simulink model "evaluateDis2009b"  (Simulink 7.4)
settings: Solver=ode45  SolverMode=SingleTasking  StartTime=0.0  StopTime=0.4  RelTol=1e-3
values from neighbouring files (symbols this model uses):
  plant = tf(1,[0.01 1])    [transferfunDisObserver_sim.m]
settings Model: Creator=Yu  LastModifiedBy=Yu  CovMetricSettings=dwe  CovHtmlReporting=off  covSaveCumulativeToWorkspaceVar=off  CovSaveSingleToWorkspaceVar=off  CovExternalEMLEnable=on
settings DataIOCC: LimitDataPoints=off  SaveFormat=StructureWithTime
settings OptimizationCC: ExpressionDepthLimit=128
settings DebuggingCC: UnderspecifiedInitializationDetection=Simplified  MergeDetectMultiDrivingBlocksExec=error  SolverPrmCheckMsg=none  FcnCallInpInsideContextMsg=Enable All  StateNameClashWarn=none  StrictBusMsg=ErrorLevel1
settings HardwareCC: ProdIntDivRoundTo=Zero  ProdEndianess=LittleEndian  ProdHWDeviceType=Specified
settings CodeAppCC: CustomSymbolStrType=$N$R$M_T
settings GRTTargetCC: TargetFunctionLibrary=C99 (ISO)  GeneratePreprocessorConditionals=Use local settings

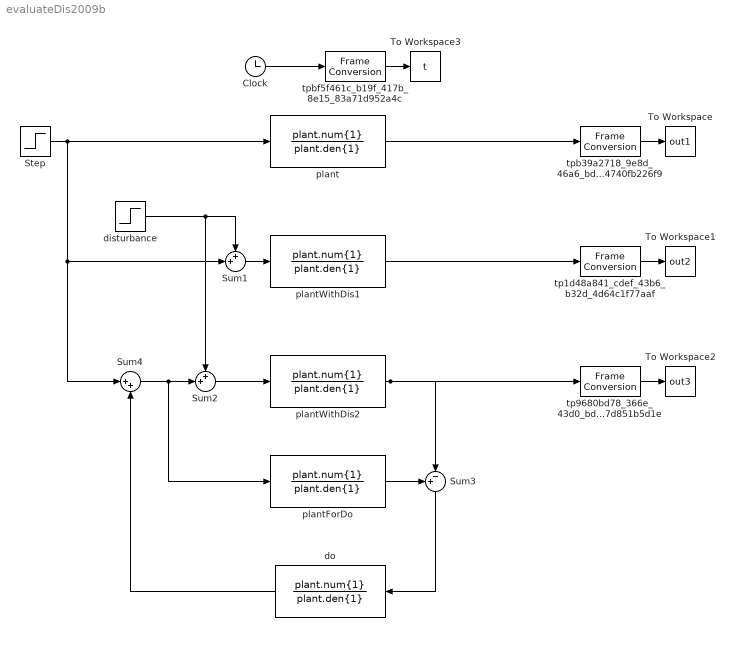
== system evaluateDis2009b ==
  Clock : Clock
  Step : Step  Time=0.01  SampleTime=0
  Sum1 : Sum  Inputs=++|
  Sum2 : Sum  Inputs=++|
  Sum3 : Sum  Inputs=+-|
  Sum4 : Sum  Inputs=|++
  To Workspace : ToWorkspace  VariableName=out1  SampleTime=-1
  To Workspace1 : ToWorkspace  VariableName=out2  SampleTime=-1
  To Workspace2 : ToWorkspace  VariableName=out3  SampleTime=-1
  To Workspace3 : ToWorkspace  VariableName=t  SampleTime=-1
  disturbance : Step  Time=0.2  After=0.3  SampleTime=0
  do : TransferFcn  Numerator=plant.num{1}  Denominator=plant.den{1}
  plant : TransferFcn  Numerator=plant.num{1}  Denominator=plant.den{1}
  plantForDo : TransferFcn  Numerator=plant.num{1}  Denominator=plant.den{1}
  plantWithDis1 : TransferFcn  Numerator=plant.num{1}  Denominator=plant.den{1}
  plantWithDis2 : TransferFcn  Numerator=plant.num{1}  Denominator=plant.den{1}
  tp1d48a841_cdef_43b6_b32d_4d64c1f77aaf : FrameConversion  InheritSamplingMode=off  OutFrame=Sample-based
  tp9680bd78_366e_43d0_bd56_b27d851b5d1e : FrameConversion  InheritSamplingMode=off  OutFrame=Sample-based
  tpb39a2718_9e8d_46a6_bd99_f4740fb226f9 : FrameConversion  InheritSamplingMode=off  OutFrame=Sample-based
  tpbf5f461c_b19f_417b_8e15_83a71d952a4c : FrameConversion  InheritSamplingMode=off  OutFrame=Sample-based
  wires:
  Step/1 -> plant/1, Sum4/1, Sum1/2
  Sum1/1 -> plantWithDis1/1
  Sum2/1 -> plantWithDis2/1
  disturbance/1 -> Sum2/1, Sum1/1
  plantForDo/1 -> Sum3/1
  plantWithDis2/1 -> Sum3/2, tp9680bd78_366e_43d0_bd56_b27d851b5d1e/1
  Sum3/1 -> do/1
  Sum4/1 -> plantForDo/1, Sum2/2
  do/1 -> Sum4/2
  plant/1 -> tpb39a2718_9e8d_46a6_bd99_f4740fb226f9/1
  tpb39a2718_9e8d_46a6_bd99_f4740fb226f9/1 -> To Workspace/1
  plantWithDis1/1 -> tp1d48a841_cdef_43b6_b32d_4d64c1f77aaf/1
  tp1d48a841_cdef_43b6_b32d_4d64c1f77aaf/1 -> To Workspace1/1
  tp9680bd78_366e_43d0_bd56_b27d851b5d1e/1 -> To Workspace2/1
  Clock/1 -> tpbf5f461c_b19f_417b_8e15_83a71d952a4c/1
  tpbf5f461c_b19f_417b_8e15_83a71d952a4c/1 -> To Workspace3/1
